simulink model "charges_pneus"  (R2024b)
settings: Solver=FixedStepAuto  StartTime=0.0  StopTime=10.0  FixedStep=Ts  RelTol=1e-3
values from neighbouring files (symbols this model uses):
  fr = 0.55    [main_data_vehicle.m]
  g = 9.81    [main_data_vehicle.m]
  h = 0.35    [main_data_vehicle.m]
  L = 1.57    [main_data_vehicle.m]
  m = 240    [main_data_vehicle.m]
settings Model: Creator=marti  LastModifiedBy=marti

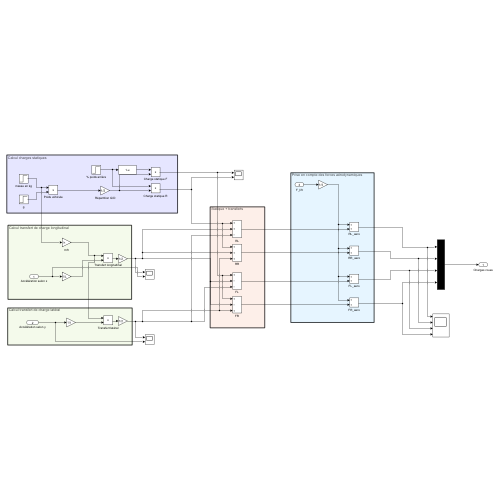
[thumbnail: Simulink's stored preview of the top-level diagram]
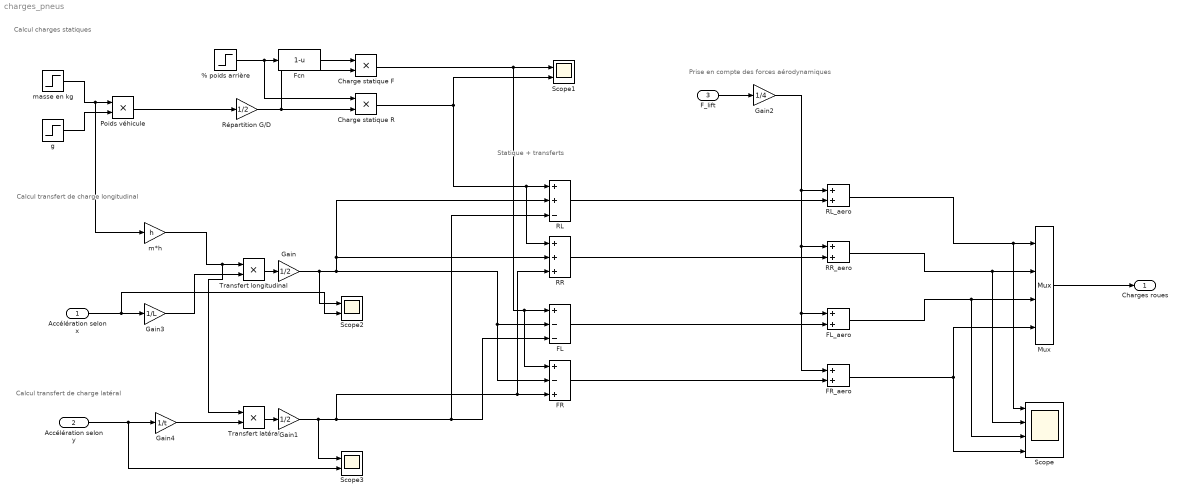
== system charges_pneus ==
  note: Prise en compte des forces aérodynamiques
  note: Statique + transferts
  note: Calcul transfert de charge latéral
  note: Calcul transfert de charge longitudinal
  note: Calcul charges statiques
  Accélération selon x : Inport
  Accélération selon y : Inport  Port=2
  F_lift : Inport  Port=3
  % poids arrière : Step  Time=0  After=fr  SampleTime=0
  Charge statique F : Product
  Charge statique R : Product
  FL : Sum  Inputs=+--
  FL_aero : Sum
  FR : Sum  Inputs=+-+
  FR_aero : Sum
  Fcn : Fcn  Expr=1-u
  Gain : Gain  Gain=1/2
  Gain1 : Gain  Gain=1/2
  Gain2 : Gain  Gain=1/4
  Gain3 : Gain  Gain=1/L
  Gain4 : Gain  Gain=1/t
  Mux : Mux
  Poids véhicule : Product
  RL : Sum  Inputs=++-
  RL_aero : Sum
  RR : Sum  Inputs=+++
  RR_aero : Sum
  Répartition G/D : Gain  Gain=1/2
  Scope : Scope  NumInputPorts=4
  Scope1 : Scope  NumInputPorts=2
  Scope2 : Scope  NumInputPorts=2
  Scope3 : Scope  NumInputPorts=2
  Transfert latéral : Product
  Transfert longitudinal : Product
  g : Step  Time=0  After=g  SampleTime=0
  m*h : Gain  Gain=h
  masse en kg : Step  Time=0  After=m  SampleTime=0
  Charges roues : Outport
  wires:
  g/1 -> Poids véhicule/2
  masse en kg/1 -> m*h/1, Poids véhicule/1
  Poids véhicule/1 -> Répartition G/D/1
  % poids arrière/1 -> Charge statique R/1, Fcn/1
  Fcn/1 -> Charge statique F/1
  Répartition G/D/1 -> Charge statique F/2, Charge statique R/2
  Accélération selon x/1 -> Gain3/1, Scope2/2
  Gain3/1 -> Transfert longitudinal/2
  m*h/1 -> Transfert latéral/1, Transfert longitudinal/1
  Accélération selon y/1 -> Gain4/1, Scope3/2
  Gain4/1 -> Transfert latéral/2
  Transfert latéral/1 -> Gain1/1
  Transfert longitudinal/1 -> Gain/1
  Charge statique F/1 -> FR/1, FL/1, Scope1/1
  Charge statique R/1 -> RR/1, RL/1, Scope1/2
  RL/1 -> RL_aero/2
  RR/1 -> RR_aero/2
  FL/1 -> FL_aero/2
  FR/1 -> FR_aero/2
  F_lift/1 -> Gain2/1
  Gain2/1 -> FR_aero/1, FL_aero/1, RR_aero/1, RL_aero/1
  RL_aero/1 -> Scope/1, Mux/1
  RR_aero/1 -> Scope/2, Mux/2
  FL_aero/1 -> Scope/3, Mux/3
  FR_aero/1 -> Scope/4, Mux/4
  Mux/1 -> Charges roues/1
  Gain/1 -> Scope2/1, FR/2, FL/2, RR/2, RL/2
  Gain1/1 -> Scope3/1, RL/3, FL/3, RR/3, FR/3
